simulink model "sampleModel7126_pp_1_1"  (R2018a)
settings: Solver=VariableStepAuto  StartTime=0.0  StopTime=10.0  RelTol=1e-3
undefined symbols (not defined in the file): DiscIntNeverNeededParam
libraries: simulink x367
(part 7 of 12)

== system sampleModel7126_pp_1_1/cfblk249/cfblk10 ==
  emi_1784 : Inport
  emi_1785 : Inport  Port=2
  Action Port : ActionPort  ActionType=then
  cfblk10 : simulink/Continuous/PID Controller (2DOF)  Controller=PID  TimeDomain=Discrete-time  SampleTime=-1  IntegratorMethod=Forward Euler  FilterMethod=Forward Euler  Form=Parallel  UseFilter=on  ControllerParametersSource=internal  P=1  I=1  D=0  N=100  b=1  c=1  InitialConditionSource=internal  InitialConditionForIntegrator=0  InitialConditionForFilter=0  ExternalReset=none  LimitOutput=off  UpperSaturationLimit=inf  LowerSaturationLimit=-inf  LinearizeAsGain=off  AntiWindupMode=none  Kb=1  TrackingMode=off  Kt=1  PParamMin=[]  PParamMax=[]  IParamMin=[]  IParamMax=[]  DParamMin=[]  DParamMax=[]  NParamMin=[]  NParamMax=[]  bParamMin=[]  bParamMax=[]  cParamMin=[]  cParamMax=[]  KbParamMin=[]  KbParamMax=[]  KtParamMin=[]  KtParamMax=[]  POutMin=[]  POutMax=[]  IOutMin=[]  IOutMax=[]  DOutMin=[]  DOutMax=[]  NOutMin=[]  NOutMax=[]  bOutMin=[]  bOutMax=[]  cOutMin=[]  cOutMax=[]  KbOutMin=[]  KbOutMax=[]  KtOutMin=[]  KtOutMax=[]  IntegratorOutMin=[]  IntegratorOutMax=[]  FilterOutMin=[]  FilterOutMax=[]  SumOutMin=[]  SumOutMax=[]  Sum1OutMin=[]  Sum1OutMax=[]  Sum2OutMin=[]  Sum2OutMax=[]  Sum3OutMin=[]  Sum3OutMax=[]  SumI1OutMin=[]  SumI1OutMax=[]  SumI2OutMin=[]  SumI2OutMax=[]  SumI3OutMin=[]  SumI3OutMax=[]  SumDOutMin=[]  SumDOutMax=[]  SaturationOutMin=[]  SaturationOutMax=[]  IntegratorContinuousStateAttributes=''  IntegratorStateMustResolveToSignalObject=off  IntegratorRTWStateStorageClass=Auto  FilterContinuousStateAttributes=''  FilterStateMustResolveToSignalObject=off  FilterRTWStateStorageClass=Auto  DifferentiatorICPrevScaledInput=0  DifferentiatorOutMin=[]  DifferentiatorOutMax=[]  FilterDiffOutCoefMin=[]  FilterDiffOutCoefMax=[]  SumDenOutMin=[]  SumDenOutMax=[]  SumNumOutMin=[]  SumNumOutMax=[]  ReciprocalOutMin=[]  ReciprocalOutMax=[]  DivideOutMin=[]  DivideOutMax=[]  TunerSelectOption=Transfer Function Based (PID Tuner App)
  emi_1786 : Outport
  wires:
  emi_1784/1 -> cfblk10/1
  emi_1785/1 -> cfblk10/2
  cfblk10/1 -> emi_1786/1

== system sampleModel7126_pp_1_1/cfblk249/cfblk3 ==
  emi_2116 : Inport
  Action Port : ActionPort  ActionType=then
  cfblk3 : DiscreteZeroPole  Poles=[0 0.5]  Gain=1  SampleTime=-1
  emi_2117 : Outport
  wires:
  emi_2116/1 -> cfblk3/1
  cfblk3/1 -> emi_2117/1

== system sampleModel7126_pp_1_1/cfblk249/cfblk5 ==
  emi_542 : Inport
  Action Port : ActionPort  ActionType=then
  cfblk5 : UnitDelay  SampleTime=-1
  emi_543 : Outport
  wires:
  emi_542/1 -> cfblk5/1
  cfblk5/1 -> emi_543/1

== system sampleModel7126_pp_1_1/cfblk249/cfblk9 ==
  emi_577 : Inport
  Action Port : ActionPort  ActionType=then
  cfblk9 : DiscreteFir
  emi_578 : Outport
  wires:
  emi_577/1 -> cfblk9/1
  cfblk9/1 -> emi_578/1

== system sampleModel7126_pp_1_1/cfblk249/emi_1787 ==
  Action Port : ActionPort  ActionType=else
  emi_1788 : Assertion

== system sampleModel7126_pp_1_1/cfblk249/emi_2118 ==
  Action Port : ActionPort  ActionType=else
  emi_2119 : Assertion

== system sampleModel7126_pp_1_1/cfblk249/emi_544 ==
  Action Port : ActionPort  ActionType=else
  emi_545 : Assertion

== system sampleModel7126_pp_1_1/cfblk249/emi_579 ==
  Action Port : ActionPort  ActionType=else
  emi_580 : Assertion

== system sampleModel7126_pp_1_1/cfblk250/cfblk4 ==
  emi_1841 : Inport
  Action Port : ActionPort  ActionType=then
  cfblk4 : simulink/Discrete/Transfer Fcn Real Zero  ZeroZ=0.75  ICPrevInput=0.0  DoSatur=off
      settings: SourceProductName=Simulink  SourceProductBaseCode=SL
  emi_1842 : Outport
  wires:
  emi_1841/1 -> cfblk4/1
  cfblk4/1 -> emi_1842/1

== system sampleModel7126_pp_1_1/cfblk250/cfblk6 ==
  emi_1313 : Inport
  Action Port : ActionPort  ActionType=then
  cfblk6 : DiscreteFir
  emi_1314 : Outport
  wires:
  emi_1313/1 -> cfblk6/1
  cfblk6/1 -> emi_1314/1

== system sampleModel7126_pp_1_1/cfblk250/emi_1315 ==
  Action Port : ActionPort  ActionType=else
  emi_1316 : Assertion

== system sampleModel7126_pp_1_1/cfblk250/emi_1843 ==
  Action Port : ActionPort  ActionType=else
  emi_1844 : Assertion

== system sampleModel7126_pp_1_1/cfblk251/cfblk5 ==
  emi_1490 : Inport
  Action Port : ActionPort  ActionType=then
  cfblk5 : simulink/Discrete/Transfer Fcn Real Zero  ZeroZ=0.75  ICPrevInput=0.0  DoSatur=off
      settings: SourceProductName=Simulink  SourceProductBaseCode=SL
  emi_1491 : Outport
  wires:
  emi_1490/1 -> cfblk5/1
  cfblk5/1 -> emi_1491/1

== system sampleModel7126_pp_1_1/cfblk251/cfblk6 ==
  emi_1398 : Inport
  Action Port : ActionPort  ActionType=then
  cfblk6 : simulink/Discrete/Transfer Fcn Lead or Lag  PoleZ=0.95  ZeroZ=0.75  ICPrevOutput=0.0  ICPrevInput=0.0  DoSatur=off
      settings: SourceProductName=Simulink  SourceProductBaseCode=SL
  emi_1399 : Outport
  wires:
  emi_1398/1 -> cfblk6/1
  cfblk6/1 -> emi_1399/1

== system sampleModel7126_pp_1_1/cfblk251/emi_1400 ==
  Action Port : ActionPort  ActionType=else
  emi_1401 : Assertion

== system sampleModel7126_pp_1_1/cfblk251/emi_1492 ==
  Action Port : ActionPort  ActionType=else
  emi_1493 : Assertion

== system sampleModel7126_pp_1_1/cfblk252/cfblk10 ==
  emi_1059 : Inport
  Action Port : ActionPort  ActionType=then
  cfblk10 : simulink/Discrete/Tapped Delay  vinit=0.0  samptime=-1  NumDelays=1  DelayOrder=Oldest  includeCurrent=off
  emi_1060 : Outport
  wires:
  emi_1059/1 -> cfblk10/1
  cfblk10/1 -> emi_1060/1

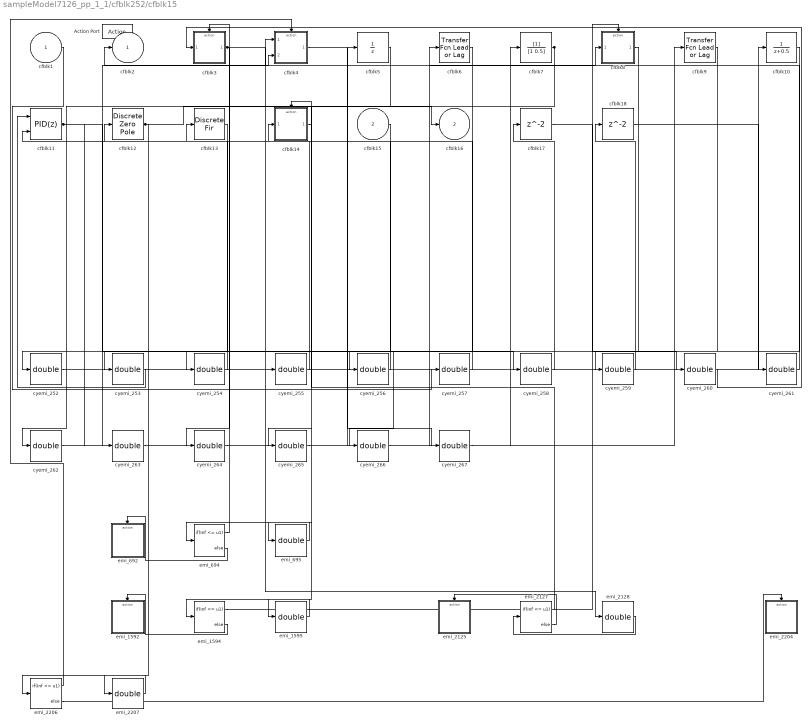
== system sampleModel7126_pp_1_1/cfblk252/cfblk15 ==
  cfblk1 : Inport
  cfblk15 : Inport  Port=2
  Action Port : ActionPort  ActionType=then
  cfblk10 : DiscreteTransferFcn
  cfblk11 : simulink/Continuous/PID Controller (2DOF)  Controller=PID  TimeDomain=Discrete-time  SampleTime=-1  IntegratorMethod=Forward Euler  FilterMethod=Forward Euler  Form=Parallel  UseFilter=on  ControllerParametersSource=internal  P=1  I=1  D=0  N=100  b=1  c=1  InitialConditionSource=internal  InitialConditionForIntegrator=0  InitialConditionForFilter=0  ExternalReset=none  LimitOutput=off  UpperSaturationLimit=inf  LowerSaturationLimit=-inf  LinearizeAsGain=off  AntiWindupMode=none  Kb=1  TrackingMode=off  Kt=1  PParamMin=[]  PParamMax=[]  IParamMin=[]  IParamMax=[]  DParamMin=[]  DParamMax=[]  NParamMin=[]  NParamMax=[]  bParamMin=[]  bParamMax=[]  cParamMin=[]  cParamMax=[]  KbParamMin=[]  KbParamMax=[]  KtParamMin=[]  KtParamMax=[]  POutMin=[]  POutMax=[]  IOutMin=[]  IOutMax=[]  DOutMin=[]  DOutMax=[]  NOutMin=[]  NOutMax=[]  bOutMin=[]  bOutMax=[]  cOutMin=[]  cOutMax=[]  KbOutMin=[]  KbOutMax=[]  KtOutMin=[]  KtOutMax=[]  IntegratorOutMin=[]  IntegratorOutMax=[]  FilterOutMin=[]  FilterOutMax=[]  SumOutMin=[]  SumOutMax=[]  Sum1OutMin=[]  Sum1OutMax=[]  Sum2OutMin=[]  Sum2OutMax=[]  Sum3OutMin=[]  Sum3OutMax=[]  SumI1OutMin=[]  SumI1OutMax=[]  SumI2OutMin=[]  SumI2OutMax=[]  SumI3OutMin=[]  SumI3OutMax=[]  SumDOutMin=[]  SumDOutMax=[]  SaturationOutMin=[]  SaturationOutMax=[]  IntegratorContinuousStateAttributes=''  IntegratorStateMustResolveToSignalObject=off  IntegratorRTWStateStorageClass=Auto  FilterContinuousStateAttributes=''  FilterStateMustResolveToSignalObject=off  FilterRTWStateStorageClass=Auto  DifferentiatorICPrevScaledInput=0  DifferentiatorOutMin=[]  DifferentiatorOutMax=[]  FilterDiffOutCoefMin=[]  FilterDiffOutCoefMax=[]  SumDenOutMin=[]  SumDenOutMax=[]  SumNumOutMin=[]  SumNumOutMax=[]  ReciprocalOutMin=[]  ReciprocalOutMax=[]  DivideOutMin=[]  DivideOutMax=[]  TunerSelectOption=Transfer Function Based (PID Tuner App)
  cfblk12 : DiscreteZeroPole  Poles=[0 0.5]  Gain=1  SampleTime=-1
  cfblk13 : DiscreteFir
  cfblk14 : Subsystem  TreatAsAtomicUnit=on
  cfblk17 : Delay
  cfblk18 : Delay
  cfblk3 : Subsystem  TreatAsAtomicUnit=on
  cfblk4 : Subsystem  TreatAsAtomicUnit=on
  cfblk5 : UnitDelay  SampleTime=-1
  cfblk6 : simulink/Discrete/Transfer Fcn Lead or Lag  PoleZ=0.95  ZeroZ=0.75  ICPrevOutput=0.0  ICPrevInput=0.0  DoSatur=off
      settings: SourceProductName=Simulink  SourceProductBaseCode=SL
  cfblk7 : DiscreteFilter
  cfblk8 : Subsystem  TreatAsAtomicUnit=on
  cfblk9 : simulink/Discrete/Transfer Fcn Lead or Lag  PoleZ=0.95  ZeroZ=0.75  ICPrevOutput=0.0  ICPrevInput=0.0  DoSatur=off
      settings: SourceProductName=Simulink  SourceProductBaseCode=SL
  cyemi_{252..267} (16 alike) : DataTypeConversion  OutDataTypeStr=double
  emi_1592 : Subsystem  TreatAsAtomicUnit=on
  emi_{694,1594,2127,2206} (4 alike) : If  IfExpression=Inf <= u1  SampleTime=[1 0]
  emi_{695,1595,2128,2207} (4 alike) : DataTypeConversion  OutDataTypeStr=double
  emi_2125 : Subsystem  TreatAsAtomicUnit=on
  emi_2204 : Subsystem  TreatAsAtomicUnit=on
  emi_692 : Subsystem  TreatAsAtomicUnit=on
  cfblk2 : Outport
  cfblk16 : Outport  Port=2
  wires:
  cfblk11/1 -> cyemi_258/1, cyemi_263/1
  cfblk12/1 -> cfblk16/1, emi_2207/1
  cfblk7/1 -> cfblk2/1, emi_695/1, emi_1595/1
  cyemi_252/1 -> cfblk10/1
  cfblk9/1 -> cyemi_252/1
  cyemi_253/1 -> cfblk11/1
  cfblk13/1 -> cyemi_253/1
  cyemi_254/1 -> cfblk11/2
  cyemi_255/1 -> cfblk12/1
  cyemi_256/1 -> cfblk13/1
  cfblk6/1 -> cyemi_256/1
  cfblk1/1 -> cyemi_257/1
  cyemi_258/1 -> cfblk17/1
  cyemi_259/1 -> cfblk18/1
  cfblk17/1 -> cyemi_260/1
  cfblk18/1 -> cyemi_261/1
  cfblk5/1 -> cyemi_262/1
  cyemi_263/1 -> cfblk5/1
  cyemi_264/1 -> cfblk6/1
  cfblk15/1 -> cyemi_264/1
  cyemi_265/1 -> cfblk7/1
  cfblk10/1 -> cyemi_266/1
  cyemi_267/1 -> cfblk9/1
  cyemi_260/1 -> cfblk3/1(emi_690)
  cfblk3/1(emi_691) -> cyemi_255/1, cyemi_254/1, emi_2128/1
  emi_694/1 -> cfblk3/Action
  emi_694/2 -> emi_692/Action
  emi_695/1 -> emi_694/1
  cyemi_266/1 -> cfblk8/1(emi_1590)
  cfblk8/1(emi_1591) -> cyemi_259/1
  emi_1594/1 -> cfblk8/Action
  emi_1594/2 -> emi_1592/Action
  emi_1595/1 -> emi_1594/1
  cyemi_257/1 -> cfblk14/1(emi_2123)
  cfblk14/1(emi_2124) -> cyemi_265/1
  emi_2127/1 -> cfblk14/Action
  emi_2127/2 -> emi_2125/Action
  emi_2128/1 -> emi_2127/1
  cyemi_261/1 -> cfblk4/1(emi_2201)
  cyemi_262/1 -> cfblk4/2(emi_2202)
  cfblk4/1(emi_2203) -> cyemi_267/1
  emi_2206/1 -> cfblk4/Action
  emi_2206/2 -> emi_2204/Action
  emi_2207/1 -> emi_2206/1

== system sampleModel7126_pp_1_1/cfblk252/cfblk16 ==
  cfblk1 : Inport
  cfblk16 : Inport  Port=2
  Action Port : ActionPort  ActionType=else
  cfblk10 : simulink/Discrete/Difference  ICPrevInput=0.0  OutMin=[]  OutMax=[]  OutDataTypeStr=double  OutputDataTypeScalingMode=double  OutDataType=fixdt(1, 16)  OutScaling=2^-10  DoSatur=off
  cfblk11 : DiscreteIntegrator  SampleTime=-1  OutDataTypeStr=double  ICPrevOutput=DiscIntNeverNeededParam  ICPrevScaledInput=DiscIntNeverNeededParam
  cfblk12 : simulink/Discrete/Transfer Fcn Real Zero  ZeroZ=0.75  ICPrevInput=0.0  DoSatur=off
      settings: SourceProductName=Simulink  SourceProductBaseCode=SL
  cfblk13 : Subsystem  TreatAsAtomicUnit=on
  cfblk14 : Delay  DelayLengthSource=Input port
      settings: InputPortMap=u0,p1
  cfblk15 : DiscreteFilter
  cfblk3 : Subsystem  TreatAsAtomicUnit=on
  cfblk4 : simulink/Discrete/Tapped Delay  vinit=0.0  samptime=-1  NumDelays=1  DelayOrder=Oldest  includeCurrent=off
  cfblk5 : simulink/Discrete/Transfer Fcn Lead or Lag  PoleZ=0.95  ZeroZ=0.75  ICPrevOutput=0.0  ICPrevInput=0.0  DoSatur=off
      settings: SourceProductName=Simulink  SourceProductBaseCode=SL
  cfblk6 : Delay  ShowEnablePort=on
      settings: InputPortMap=u0,e6
  cfblk7 : Subsystem  TreatAsAtomicUnit=on
  cfblk8 : simulink/Discrete/Transfer Fcn Lead or Lag  PoleZ=0.95  ZeroZ=0.75  ICPrevOutput=0.0  ICPrevInput=0.0  DoSatur=off
      settings: SourceProductName=Simulink  SourceProductBaseCode=SL
  cfblk9 : UnitDelay  SampleTime=-1
  cyemi_{270..285} (16 alike) : DataTypeConversion  OutDataTypeStr=double
  emi_1097 : Subsystem  TreatAsAtomicUnit=on
  emi_1099 : If  IfExpression=0 <= u1  SampleTime=[1 0]
  emi_1100 : DataTypeConversion  OutDataTypeStr=double
  emi_112 : Subsystem  TreatAsAtomicUnit=on
  emi_114 : If  IfExpression=0 <= u1  SampleTime=[1 0]
  emi_115 : DataTypeConversion  OutDataTypeStr=double
  emi_261 : Subsystem  TreatAsAtomicUnit=on
  emi_263 : If  IfExpression=0 <= u1  SampleTime=[1 0]
  emi_264 : DataTypeConversion  OutDataTypeStr=double
  cfblk2 : Outport
  cfblk17 : Outport  Port=2
  wires:
  cfblk8/1 -> cyemi_270/1, cyemi_281/1
  cfblk9/1 -> cfblk2/1
  cyemi_270/1 -> cfblk10/1
  cyemi_271/1 -> cfblk11/1
  cfblk4/1 -> cyemi_271/1, emi_115/1
  cyemi_272/1 -> cfblk12/1
  cfblk10/1 -> cyemi_273/1
  cyemi_274/1 -> cfblk14/1
  cfblk15/1 -> cyemi_274/1, cyemi_275/1
  cyemi_275/1 -> cfblk14/2
  cyemi_276/1 -> cfblk15/1
  cfblk5/1 -> cyemi_276/1
  cfblk14/1 -> cyemi_277/1
  cfblk16/1 -> cyemi_278/1
  cyemi_279/1 -> cfblk4/1
  cyemi_280/1 -> cfblk5/1
  cyemi_281/1 -> cfblk6/1
  cyemi_282/1 -> cfblk6/2
  cfblk12/1 -> cyemi_282/1
  cfblk1/1 -> cyemi_283/1
  cyemi_284/1 -> cfblk8/1
  cfblk11/1 -> cyemi_284/1
  cyemi_285/1 -> cfblk9/1
  cfblk6/1 -> cyemi_285/1
  cyemi_277/1 -> cfblk3/1(emi_109)
  cyemi_278/1 -> cfblk3/2(emi_110)
  cfblk3/1(emi_111) -> cyemi_279/1, emi_264/1, emi_1100/1
  emi_114/1 -> cfblk3/Action
  emi_114/2 -> emi_112/Action
  emi_115/1 -> emi_114/1
  cyemi_273/1 -> cfblk13/1(emi_259)
  cfblk13/1(emi_260) -> cyemi_272/1, cfblk17/1
  emi_263/1 -> cfblk13/Action
  emi_263/2 -> emi_261/Action
  emi_264/1 -> emi_263/1
  cyemi_283/1 -> cfblk7/1(emi_1095)
  cfblk7/1(emi_1096) -> cyemi_280/1
  emi_1099/1 -> cfblk7/Action
  emi_1099/2 -> emi_1097/Action
  emi_1100/1 -> emi_1099/1

== system sampleModel7126_pp_1_1/cfblk252/cfblk7 ==
  emi_166 : Inport
  Action Port : ActionPort  ActionType=then
  cfblk7 : UnitDelay  SampleTime=-1
  emi_167 : Outport
  wires:
  emi_166/1 -> cfblk7/1
  cfblk7/1 -> emi_167/1

== system sampleModel7126_pp_1_1/cfblk252/cfblk8 ==
  emi_2080 : Inport
  Action Port : ActionPort  ActionType=then
  cfblk8 : simulink/Discrete/Difference  ICPrevInput=0.0  OutMin=[]  OutMax=[]  OutDataTypeStr=double  OutputDataTypeScalingMode=double  OutDataType=fixdt(1, 16)  OutScaling=2^-10  DoSatur=off
  emi_2081 : Outport
  wires:
  emi_2080/1 -> cfblk8/1
  cfblk8/1 -> emi_2081/1

== system sampleModel7126_pp_1_1/cfblk252/emi_1061 ==
  Action Port : ActionPort  ActionType=else
  emi_1062 : Assertion

== system sampleModel7126_pp_1_1/cfblk252/emi_168 ==
  Action Port : ActionPort  ActionType=else
  emi_169 : Assertion

== system sampleModel7126_pp_1_1/cfblk252/emi_2082 ==
  Action Port : ActionPort  ActionType=else
  emi_2083 : Assertion

== system sampleModel7126_pp_1_1/cfblk253/cfblk10 ==
  cfblk1 : Inport
  cfblk12 : Inport  Port=2
  cfblk13 : Inport  Port=3
  cfblk14 : Inport  Port=4
  Action Port : ActionPort  ActionType=else
  cfblk10 : DiscreteFilter
  cfblk11 : Subsystem  TreatAsAtomicUnit=on
  cfblk3 : simulink/Discrete/Transfer Fcn First Order  PoleZ=0.95  ICPrevOutput=0.0  DoSatur=off
      settings: SourceProductName=Simulink
  cfblk4 : simulink/Discrete/Difference  ICPrevInput=0.0  OutMin=[]  OutMax=[]  OutDataTypeStr=double  OutputDataTypeScalingMode=double  OutDataType=fixdt(1, 16)  OutScaling=2^-10  DoSatur=off
  cfblk5 : DiscreteStateSpace  SampleTime=-1
  cfblk6 : Delay
  cfblk7 : DiscreteZeroPole  Poles=[0 0.5]  Gain=1  SampleTime=-1
  cfblk8 : Delay
  cfblk9 : UnitDelay  SampleTime=-1
  cyemi_{303..311} (9 alike) : DataTypeConversion  OutDataTypeStr=double
  emi_2111 : Subsystem  TreatAsAtomicUnit=on
  emi_2113 : If  IfExpression=0 <= u1  SampleTime=[1 0]
  emi_2114 : DataTypeConversion  OutDataTypeStr=double
  cfblk2 : Outport
  cfblk15 : Outport  Port=2
  wires:
  cfblk3/1 -> cfblk2/1
  cfblk12/1 -> cfblk15/1
  cyemi_303/1 -> cfblk10/1
  cfblk8/1 -> cyemi_303/1
  cfblk10/1 -> cyemi_304/1
  cyemi_305/1 -> cfblk3/1
  cfblk7/1 -> cyemi_305/1
  cyemi_306/1 -> cfblk4/1
  cfblk5/1 -> cyemi_306/1, emi_2114/1
  cyemi_307/1 -> cfblk5/1
  cfblk14/1 -> cyemi_307/1
  cyemi_308/1 -> cfblk6/1
  cfblk1/1 -> cyemi_308/1
  cyemi_309/1 -> cfblk7/1
  cyemi_310/1 -> cfblk8/1
  cfblk13/1 -> cyemi_310/1
  cyemi_311/1 -> cfblk9/1
  cfblk4/1 -> cyemi_311/1
  cyemi_304/1 -> cfblk11/1(emi_2109)
  cfblk11/1(emi_2110) -> cyemi_309/1
  emi_2113/1 -> cfblk11/Action
  emi_2113/2 -> emi_2111/Action
  emi_2114/1 -> emi_2113/1

== system sampleModel7126_pp_1_1/cfblk253/cfblk15 ==
  emi_711 : Inport
  Action Port : ActionPort  ActionType=then
  cfblk15 : Delay
  emi_712 : Outport
  wires:
  emi_711/1 -> cfblk15/1
  cfblk15/1 -> emi_712/1

== system sampleModel7126_pp_1_1/cfblk253/cfblk4 ==
  emi_1497 : Inport
  Action Port : ActionPort  ActionType=then
  cfblk4 : simulink/Discrete/Transfer Fcn Real Zero  ZeroZ=0.75  ICPrevInput=0.0  DoSatur=off
      settings: SourceProductName=Simulink  SourceProductBaseCode=SL
  emi_1498 : Outport
  wires:
  emi_1497/1 -> cfblk4/1
  cfblk4/1 -> emi_1498/1

== system sampleModel7126_pp_1_1/cfblk253/cfblk9 ==
  cfblk1 : Inport
  cfblk4 : Inport  Port=2
  cfblk5 : Inport  Port=3
  cfblk6 : Inport  Port=4
  Action Port : ActionPort  ActionType=then
  cfblk3 : DiscreteZeroPole  Poles=[0 0.5]  Gain=1  SampleTime=-1
  cyemi_327 : DataTypeConversion  OutDataTypeStr=double
  cfblk2 : Outport
  cfblk7 : Outport  Port=2
  cfblk8 : Outport  Port=3
  cfblk9 : Outport  Port=4
  wires:
  cfblk1/1 -> cfblk2/1
  cfblk6/1 -> cfblk8/1
  cfblk5/1 -> cfblk7/1
  cfblk3/1 -> cfblk9/1
  cyemi_327/1 -> cfblk3/1
  cfblk4/1 -> cyemi_327/1

== system sampleModel7126_pp_1_1/cfblk253/emi_1499 ==
  Action Port : ActionPort  ActionType=else
  emi_1500 : Assertion

== system sampleModel7126_pp_1_1/cfblk253/emi_713 ==
  Action Port : ActionPort  ActionType=else
  emi_714 : Assertion

== system sampleModel7126_pp_1_1/cfblk255/cfblk3 ==
  emi_774 : Inport
  Action Port : ActionPort  ActionType=then
  cfblk3 : simulink/Discrete/Transfer Fcn Lead or Lag  PoleZ=0.95  ZeroZ=0.75  ICPrevOutput=0.0  ICPrevInput=0.0  DoSatur=off
      settings: SourceProductName=Simulink  SourceProductBaseCode=SL
  emi_775 : Outport
  wires:
  emi_774/1 -> cfblk3/1
  cfblk3/1 -> emi_775/1

== system sampleModel7126_pp_1_1/cfblk255/cfblk5 ==
  emi_1792 : Inport
  Action Port : ActionPort  ActionType=then
  cfblk5 : Delay
  emi_1793 : Outport
  wires:
  emi_1792/1 -> cfblk5/1
  cfblk5/1 -> emi_1793/1

== system sampleModel7126_pp_1_1/cfblk255/cfblk6 ==
  emi_945 : Inport
  emi_946 : Inport  Port=2
  Action Port : ActionPort  ActionType=then
  cfblk6 : Delay  ShowEnablePort=on
      settings: InputPortMap=u0,e6
  emi_947 : Outport
  wires:
  emi_945/1 -> cfblk6/1
  emi_946/1 -> cfblk6/2
  cfblk6/1 -> emi_947/1

== system sampleModel7126_pp_1_1/cfblk255/emi_1794 ==
  Action Port : ActionPort  ActionType=else
  emi_1795 : Assertion

== system sampleModel7126_pp_1_1/cfblk255/emi_776 ==
  Action Port : ActionPort  ActionType=else
  emi_777 : Assertion

== system sampleModel7126_pp_1_1/cfblk255/emi_948 ==
  Action Port : ActionPort  ActionType=else
  emi_949 : Assertion

== system sampleModel7126_pp_1_1/cfblk256/cfblk11 ==
  cfblk1 : Inport
  cfblk9 : Inport  Port=2
  cfblk10 : Inport  Port=3
  Action Port : ActionPort  ActionType=then
  cfblk3 : Subsystem  TreatAsAtomicUnit=on
  cfblk4 : simulink/Discrete/Transfer Fcn Real Zero  ZeroZ=0.75  ICPrevInput=0.0  DoSatur=off
      settings: SourceProductName=Simulink  SourceProductBaseCode=SL
  cfblk5 : DiscreteStateSpace  SampleTime=-1
  cfblk6 : DiscreteTransferFcn
  cfblk7 : Subsystem  TreatAsAtomicUnit=on
  cfblk8 : DiscreteFir
  cyemi_{362..367} (6 alike) : DataTypeConversion  OutDataTypeStr=double
  emi_1133 : Subsystem  TreatAsAtomicUnit=on
  emi_1135 : If  IfExpression=Inf <= u1
  emi_1136 : DataTypeConversion  OutDataTypeStr=double
  emi_572 : Subsystem  TreatAsAtomicUnit=on
  emi_574 : If  IfExpression=Inf <= u1  SampleTime=[1 0]
  emi_575 : DataTypeConversion  OutDataTypeStr=double
  cfblk2 : Outport
  cfblk11 : Outport  Port=2
  wires:
  cfblk6/1 -> cfblk11/1, emi_1136/1
  cfblk9/1 -> cyemi_362/1
  cyemi_363/1 -> cfblk4/1
  cfblk1/1 -> cyemi_363/1
  cyemi_364/1 -> cfblk5/1
  cfblk8/1 -> cyemi_364/1
  cyemi_365/1 -> cfblk6/1
  cfblk4/1 -> cyemi_365/1
  cfblk5/1 -> cyemi_366/1, emi_575/1
  cyemi_367/1 -> cfblk8/1
  cyemi_366/1 -> cfblk7/1(emi_570)
  cfblk7/1(emi_571) -> cfblk2/1
  emi_574/1 -> cfblk7/Action
  emi_574/2 -> emi_572/Action
  emi_575/1 -> emi_574/1
  cyemi_362/1 -> cfblk3/1(emi_1131)
  cfblk3/1(emi_1132) -> cyemi_367/1
  emi_1135/1 -> cfblk3/Action
  emi_1135/2 -> emi_1133/Action
  emi_1136/1 -> emi_1135/1

== system sampleModel7126_pp_1_1/cfblk256/cfblk12 ==
  cfblk1 : Inport
  Action Port : ActionPort  ActionType=else
  cfblk3 : DiscreteTransferFcn
  cfblk4 : simulink/Discrete/Difference  ICPrevInput=0.0  OutMin=[]  OutMax=[]  OutDataTypeStr=double  OutputDataTypeScalingMode=double  OutDataType=fixdt(1, 16)  OutScaling=2^-10  DoSatur=off
  cfblk5 : DiscreteIntegrator  SampleTime=-1  OutDataTypeStr=double  ICPrevOutput=DiscIntNeverNeededParam  ICPrevScaledInput=DiscIntNeverNeededParam
  cfblk6 : Delay
  cyemi_{369..372} (4 alike) : DataTypeConversion  OutDataTypeStr=double
  cfblk2 : Outport
  cfblk7 : Outport  Port=2
  cfblk8 : Outport  Port=3
  wires:
  cfblk4/1 -> cfblk7/1, cfblk2/1
  cfblk3/1 -> cfblk8/1, cyemi_371/1
  cyemi_369/1 -> cfblk3/1
  cfblk1/1 -> cyemi_369/1
  cyemi_370/1 -> cfblk4/1
  cfblk6/1 -> cyemi_370/1
  cyemi_371/1 -> cfblk5/1
  cyemi_372/1 -> cfblk6/1
  cfblk5/1 -> cyemi_372/1

== system sampleModel7126_pp_1_1/cfblk256/cfblk14 ==
  emi_2144 : Inport
  Action Port : ActionPort  ActionType=then
  cfblk14 : Delay
  emi_2145 : Outport
  wires:
  emi_2144/1 -> cfblk14/1
  cfblk14/1 -> emi_2145/1

== system sampleModel7126_pp_1_1/cfblk256/cfblk3 ==
  emi_1038 : Inport
  Action Port : ActionPort  ActionType=then
  cfblk3 : DiscreteTransferFcn
  emi_1039 : Outport
  wires:
  emi_1038/1 -> cfblk3/1
  cfblk3/1 -> emi_1039/1

== system sampleModel7126_pp_1_1/cfblk256/emi_1040 ==
  Action Port : ActionPort  ActionType=else
  emi_1041 : Assertion

== system sampleModel7126_pp_1_1/cfblk256/emi_2146 ==
  Action Port : ActionPort  ActionType=else
  emi_2147 : Assertion

== system sampleModel7126_pp_1_1/cfblk257/cfblk7 ==
  emi_1632 : Inport
  Action Port : ActionPort  ActionType=then
  cfblk7 : simulink/Continuous/PID Controller  Controller=PID  TimeDomain=Discrete-time  SampleTime=-1  IntegratorMethod=Forward Euler  FilterMethod=Forward Euler  Form=Parallel  UseFilter=on  ControllerParametersSource=internal  P=1  I=1  D=0  N=100  InitialConditionSource=internal  InitialConditionForIntegrator=0  InitialConditionForFilter=0  ExternalReset=none  LimitOutput=off  UpperSaturationLimit=inf  LowerSaturationLimit=-inf  LinearizeAsGain=off  AntiWindupMode=none  Kb=1  TrackingMode=off  Kt=1  PParamMin=[]  PParamMax=[]  IParamMin=[]  IParamMax=[]  DParamMin=[]  DParamMax=[]  NParamMin=[]  NParamMax=[]  KbParamMin=[]  KbParamMax=[]  KtParamMin=[]  KtParamMax=[]  POutMin=[]  POutMax=[]  IOutMin=[]  IOutMax=[]  DOutMin=[]  DOutMax=[]  NOutMin=[]  NOutMax=[]  KbOutMin=[]  KbOutMax=[]  KtOutMin=[]  KtOutMax=[]  IntegratorOutMin=[]  IntegratorOutMax=[]  FilterOutMin=[]  FilterOutMax=[]  SumOutMin=[]  SumOutMax=[]  SumI1OutMin=[]  SumI1OutMax=[]  SumI2OutMin=[]  SumI2OutMax=[]  SumI3OutMin=[]  SumI3OutMax=[]  SumDOutMin=[]  SumDOutMax=[]  SaturationOutMin=[]  SaturationOutMax=[]  IntegratorContinuousStateAttributes=''  IntegratorStateMustResolveToSignalObject=off  IntegratorRTWStateStorageClass=Auto  FilterContinuousStateAttributes=''  FilterStateMustResolveToSignalObject=off  FilterRTWStateStorageClass=Auto  DifferentiatorICPrevScaledInput=0  DifferentiatorOutMin=[]  DifferentiatorOutMax=[]  FilterDiffOutCoefMin=[]  FilterDiffOutCoefMax=[]  SumDenOutMin=[]  SumDenOutMax=[]  SumNumOutMin=[]  SumNumOutMax=[]  ReciprocalOutMin=[]  ReciprocalOutMax=[]  DivideOutMin=[]  DivideOutMax=[]  TunerSelectOption=Transfer Function Based (PID Tuner App)
  emi_1633 : Outport
  wires:
  emi_1632/1 -> cfblk7/1
  cfblk7/1 -> emi_1633/1

== system sampleModel7126_pp_1_1/cfblk257/cfblk9 ==
  emi_725 : Inport
  Action Port : ActionPort  ActionType=then
  cfblk9 : DiscreteStateSpace  SampleTime=-1
  emi_726 : Outport
  wires:
  emi_725/1 -> cfblk9/1
  cfblk9/1 -> emi_726/1

== system sampleModel7126_pp_1_1/cfblk257/emi_1634 ==
  Action Port : ActionPort  ActionType=else
  emi_1635 : Assertion

== system sampleModel7126_pp_1_1/cfblk257/emi_727 ==
  Action Port : ActionPort  ActionType=else
  emi_728 : Assertion

== system sampleModel7126_pp_1_1/cfblk258/cfblk5 ==
  emi_1341 : Inport
  Action Port : ActionPort  ActionType=then
  cfblk5 : UnitDelay  SampleTime=-1
  emi_1342 : Outport
  wires:
  emi_1341/1 -> cfblk5/1
  cfblk5/1 -> emi_1342/1

== system sampleModel7126_pp_1_1/cfblk258/emi_1343 ==
  Action Port : ActionPort  ActionType=else
  emi_1344 : Assertion

== system sampleModel7126_pp_1_1/cfblk259/cfblk10 ==
  cfblk1 : Inport
  cfblk10 : Inport  Port=2
  cfblk11 : Inport  Port=3
  cfblk12 : Inport  Port=4
  Action Port : ActionPort  ActionType=else
  cfblk13 : Subsystem  TreatAsAtomicUnit=on
  cfblk3 : DiscreteZeroPole  Poles=[0 0.5]  Gain=1  SampleTime=-1
  cfblk4 : Subsystem  TreatAsAtomicUnit=on
  cfblk5 : DiscreteStateSpace  SampleTime=-1
  cfblk6 : Subsystem  TreatAsAtomicUnit=on
  cfblk7 : DiscreteStateSpace  SampleTime=-1
  cfblk8 : simulink/Discrete/Transfer Fcn First Order  PoleZ=0.95  ICPrevOutput=0.0  DoSatur=off
      settings: SourceProductName=Simulink
  cfblk9 : Subsystem  TreatAsAtomicUnit=on
  cyemi_{412..420} (9 alike) : DataTypeConversion  OutDataTypeStr=double
  emi_1550 : Subsystem  TreatAsAtomicUnit=on
  emi_1552 : If  IfExpression=Inf <= u1  SampleTime=[1 0]
  emi_{377,816,865,1553} (4 alike) : DataTypeConversion  OutDataTypeStr=double
  emi_374 : Subsystem  TreatAsAtomicUnit=on
  emi_376 : If  IfExpression=Inf <= u1
  emi_813 : Subsystem  TreatAsAtomicUnit=on
  emi_815 : If  IfExpression=Inf <= u1  SampleTime=[1 0]
  emi_862 : Subsystem  TreatAsAtomicUnit=on
  emi_864 : If  IfExpression=Inf <= u1  SampleTime=[1 0]
  cfblk2 : Outport
  wires:
  cfblk10/1 -> cfblk2/1
  cyemi_413/1 -> cfblk3/1
  cfblk5/1 -> cyemi_413/1, emi_377/1
  cfblk12/1 -> cyemi_414/1
  cyemi_416/1 -> cfblk5/1
  cfblk11/1 -> cyemi_416/1
  cyemi_418/1 -> cfblk7/1
  cyemi_419/1 -> cfblk8/1
  cfblk3/1 -> cyemi_419/1
  cfblk1/1 -> cyemi_420/1
  cyemi_412/1 -> cfblk13/1(emi_372)
  cfblk13/1(emi_373) -> cyemi_415/1, emi_816/1, emi_865/1
  emi_376/1 -> cfblk13/Action
  emi_376/2 -> emi_374/Action
  emi_377/1 -> emi_376/1
  cyemi_417/1 -> cfblk6/1(emi_811)
  cfblk6/1(emi_812) -> cyemi_412/1, emi_1553/1
  emi_815/1 -> cfblk6/Action
  emi_815/2 -> emi_813/Action
  emi_816/1 -> emi_815/1
  cyemi_420/1 -> cfblk9/1(emi_860)
  cfblk9/1(emi_861) -> cyemi_418/1
  emi_864/1 -> cfblk9/Action
  emi_864/2 -> emi_862/Action
  emi_865/1 -> emi_864/1
  cyemi_414/1 -> cfblk4/1(emi_1547)
  cyemi_415/1 -> cfblk4/2(emi_1548)
  cfblk4/1(emi_1549) -> cyemi_417/1
  emi_1552/1 -> cfblk4/Action
  emi_1552/2 -> emi_1550/Action
  emi_1553/1 -> emi_1552/1

== system sampleModel7126_pp_1_1/cfblk259/cfblk11 ==
  emi_43 : Inport
  Action Port : ActionPort  ActionType=then
  cfblk11 : Delay
  emi_44 : Outport
  wires:
  emi_43/1 -> cfblk11/1
  cfblk11/1 -> emi_44/1

== system sampleModel7126_pp_1_1/cfblk259/cfblk13 ==
  emi_58 : Inport
  Action Port : ActionPort  ActionType=then
  cfblk13 : Delay
  emi_59 : Outport
  wires:
  emi_58/1 -> cfblk13/1
  cfblk13/1 -> emi_59/1

== system sampleModel7126_pp_1_1/cfblk259/cfblk3 ==
  emi_1769 : Inport
  emi_1770 : Inport  Port=2
  Action Port : ActionPort  ActionType=then
  cfblk3 : Delay  DelayLengthSource=Input port
      settings: InputPortMap=u0,p1
  emi_1771 : Outport
  wires:
  emi_1769/1 -> cfblk3/1
  emi_1770/1 -> cfblk3/2
  cfblk3/1 -> emi_1771/1

== system sampleModel7126_pp_1_1/cfblk259/cfblk4 ==
  emi_1159 : Inport
  Action Port : ActionPort  ActionType=then
  cfblk4 : DiscreteFir
  emi_1160 : Outport
  wires:
  emi_1159/1 -> cfblk4/1
  cfblk4/1 -> emi_1160/1

== system sampleModel7126_pp_1_1/cfblk259/cfblk6 ==
  emi_556 : Inport
  Action Port : ActionPort  ActionType=then
  cfblk6 : simulink/Continuous/PID Controller  Controller=PID  TimeDomain=Discrete-time  SampleTime=-1  IntegratorMethod=Forward Euler  FilterMethod=Forward Euler  Form=Parallel  UseFilter=on  ControllerParametersSource=internal  P=1  I=1  D=0  N=100  InitialConditionSource=internal  InitialConditionForIntegrator=0  InitialConditionForFilter=0  ExternalReset=none  LimitOutput=off  UpperSaturationLimit=inf  LowerSaturationLimit=-inf  LinearizeAsGain=off  AntiWindupMode=none  Kb=1  TrackingMode=off  Kt=1  PParamMin=[]  PParamMax=[]  IParamMin=[]  IParamMax=[]  DParamMin=[]  DParamMax=[]  NParamMin=[]  NParamMax=[]  KbParamMin=[]  KbParamMax=[]  KtParamMin=[]  KtParamMax=[]  POutMin=[]  POutMax=[]  IOutMin=[]  IOutMax=[]  DOutMin=[]  DOutMax=[]  NOutMin=[]  NOutMax=[]  KbOutMin=[]  KbOutMax=[]  KtOutMin=[]  KtOutMax=[]  IntegratorOutMin=[]  IntegratorOutMax=[]  FilterOutMin=[]  FilterOutMax=[]  SumOutMin=[]  SumOutMax=[]  SumI1OutMin=[]  SumI1OutMax=[]  SumI2OutMin=[]  SumI2OutMax=[]  SumI3OutMin=[]  SumI3OutMax=[]  SumDOutMin=[]  SumDOutMax=[]  SaturationOutMin=[]  SaturationOutMax=[]  IntegratorContinuousStateAttributes=''  IntegratorStateMustResolveToSignalObject=off  IntegratorRTWStateStorageClass=Auto  FilterContinuousStateAttributes=''  FilterStateMustResolveToSignalObject=off  FilterRTWStateStorageClass=Auto  DifferentiatorICPrevScaledInput=0  DifferentiatorOutMin=[]  DifferentiatorOutMax=[]  FilterDiffOutCoefMin=[]  FilterDiffOutCoefMax=[]  SumDenOutMin=[]  SumDenOutMax=[]  SumNumOutMin=[]  SumNumOutMax=[]  ReciprocalOutMin=[]  ReciprocalOutMax=[]  DivideOutMin=[]  DivideOutMax=[]  TunerSelectOption=Transfer Function Based (PID Tuner App)
  emi_557 : Outport
  wires:
  emi_556/1 -> cfblk6/1
  cfblk6/1 -> emi_557/1

== system sampleModel7126_pp_1_1/cfblk259/cfblk9 ==
  cfblk1 : Inport
  cfblk11 : Inport  Port=2
  Action Port : ActionPort  ActionType=then
  cfblk10 : Subsystem  TreatAsAtomicUnit=on
  cfblk14 : Subsystem  TreatAsAtomicUnit=on
  cfblk15 : Delay
  cfblk3 : simulink/Discrete/Tapped Delay  vinit=0.0  samptime=-1  NumDelays=1  DelayOrder=Oldest  includeCurrent=off
  cfblk4 : Delay  ShowEnablePort=on
      settings: InputPortMap=u0,e6
  cfblk5 : simulink/Discrete/Transfer Fcn First Order  PoleZ=0.95  ICPrevOutput=0.0  DoSatur=off
      settings: SourceProductName=Simulink
  cfblk6 : DiscreteFilter
  cfblk7 : Delay  DelayLengthSource=Input port
      settings: InputPortMap=u0,p1
  cfblk8 : Subsystem  TreatAsAtomicUnit=on
  cfblk9 : Subsystem  TreatAsAtomicUnit=on
  cyemi_{432..445} (14 alike) : DataTypeConversion  OutDataTypeStr=double
  emi_1147 : Subsystem  TreatAsAtomicUnit=on
  emi_1149 : If  IfExpression=Inf <= u1
  emi_{406,1150,1289,1897} (4 alike) : DataTypeConversion  OutDataTypeStr=double
  emi_1286 : Subsystem  TreatAsAtomicUnit=on
  emi_1288 : If  IfExpression=Inf <= u1  SampleTime=[1 0]
  emi_1894 : Subsystem  TreatAsAtomicUnit=on
  emi_1896 : If  IfExpression=Inf <= u1  SampleTime=[1 0]
  emi_403 : Subsystem  TreatAsAtomicUnit=on
  emi_405 : If  IfExpression=Inf <= u1  SampleTime=[1 0]
  cfblk2 : Outport
  cfblk12 : Outport  Port=2
  cfblk13 : Outport  Port=3
  wires:
  cfblk6/1 -> cyemi_434/1, cyemi_438/1, emi_406/1
  cfblk3/1 -> cfblk2/1, cyemi_439/1
  cfblk7/1 -> cyemi_433/1
  cyemi_434/1 -> cfblk15/1
  cyemi_435/1 -> cfblk3/1
  cyemi_436/1 -> cfblk4/1
  cyemi_437/1 -> cfblk4/2
  cyemi_438/1 -> cfblk5/1
  cyemi_439/1 -> cfblk6/1
  cyemi_440/1 -> cfblk7/1
  cfblk5/1 -> cyemi_440/1
  cyemi_441/1 -> cfblk7/2
  cfblk4/1 -> cyemi_442/1
  cfblk15/1 -> cyemi_443/1
  cfblk11/1 -> cyemi_444/1
  cfblk1/1 -> cyemi_445/1
  cyemi_442/1 -> cfblk8/1(emi_400)
  cyemi_443/1 -> cfblk8/2(emi_401)
  cfblk8/1(emi_402) -> cyemi_432/1, cfblk13/1, cfblk12/1, emi_1897/1
  emi_405/1 -> cfblk8/Action
  emi_405/2 -> emi_403/Action
  emi_406/1 -> emi_405/1
  cyemi_432/1 -> cfblk10/1(emi_1145)
  cfblk10/1(emi_1146) -> cyemi_441/1, cyemi_435/1
  emi_1149/1 -> cfblk10/Action
  emi_1149/2 -> emi_1147/Action
  emi_1150/1 -> emi_1149/1
  cyemi_444/1 -> cfblk9/1(emi_1283)
  cyemi_445/1 -> cfblk9/2(emi_1284)
  cfblk9/1(emi_1285) -> cyemi_437/1
  emi_1288/1 -> cfblk9/Action
  emi_1288/2 -> emi_1286/Action
  emi_1289/1 -> emi_1288/1
  cyemi_433/1 -> cfblk14/1(emi_1892)
  cfblk14/1(emi_1893) -> emi_1289/1, emi_1150/1, cyemi_436/1
  emi_1896/1 -> cfblk14/Action
  emi_1896/2 -> emi_1894/Action
  emi_1897/1 -> emi_1896/1

== system sampleModel7126_pp_1_1/cfblk259/emi_1161 ==
  Action Port : ActionPort  ActionType=else
  emi_1162 : Assertion

== system sampleModel7126_pp_1_1/cfblk259/emi_1772 ==
  Action Port : ActionPort  ActionType=else
  emi_1773 : Assertion

== system sampleModel7126_pp_1_1/cfblk259/emi_45 ==
  Action Port : ActionPort  ActionType=else
  emi_46 : Assertion

== system sampleModel7126_pp_1_1/cfblk259/emi_558 ==
  Action Port : ActionPort  ActionType=else
  emi_559 : Assertion

== system sampleModel7126_pp_1_1/cfblk259/emi_60 ==
  Action Port : ActionPort  ActionType=else
  emi_61 : Assertion

== system sampleModel7126_pp_1_1/cfblk260/cfblk4 ==
  emi_252 : Inport
  Action Port : ActionPort  ActionType=then
  cfblk4 : simulink/Continuous/PID Controller  Controller=PID  TimeDomain=Discrete-time  SampleTime=-1  IntegratorMethod=Forward Euler  FilterMethod=Forward Euler  Form=Parallel  UseFilter=on  ControllerParametersSource=internal  P=1  I=1  D=0  N=100  InitialConditionSource=internal  InitialConditionForIntegrator=0  InitialConditionForFilter=0  ExternalReset=none  LimitOutput=off  UpperSaturationLimit=inf  LowerSaturationLimit=-inf  LinearizeAsGain=off  AntiWindupMode=none  Kb=1  TrackingMode=off  Kt=1  PParamMin=[]  PParamMax=[]  IParamMin=[]  IParamMax=[]  DParamMin=[]  DParamMax=[]  NParamMin=[]  NParamMax=[]  KbParamMin=[]  KbParamMax=[]  KtParamMin=[]  KtParamMax=[]  POutMin=[]  POutMax=[]  IOutMin=[]  IOutMax=[]  DOutMin=[]  DOutMax=[]  NOutMin=[]  NOutMax=[]  KbOutMin=[]  KbOutMax=[]  KtOutMin=[]  KtOutMax=[]  IntegratorOutMin=[]  IntegratorOutMax=[]  FilterOutMin=[]  FilterOutMax=[]  SumOutMin=[]  SumOutMax=[]  SumI1OutMin=[]  SumI1OutMax=[]  SumI2OutMin=[]  SumI2OutMax=[]  SumI3OutMin=[]  SumI3OutMax=[]  SumDOutMin=[]  SumDOutMax=[]  SaturationOutMin=[]  SaturationOutMax=[]  IntegratorContinuousStateAttributes=''  IntegratorStateMustResolveToSignalObject=off  IntegratorRTWStateStorageClass=Auto  FilterContinuousStateAttributes=''  FilterStateMustResolveToSignalObject=off  FilterRTWStateStorageClass=Auto  DifferentiatorICPrevScaledInput=0  DifferentiatorOutMin=[]  DifferentiatorOutMax=[]  FilterDiffOutCoefMin=[]  FilterDiffOutCoefMax=[]  SumDenOutMin=[]  SumDenOutMax=[]  SumNumOutMin=[]  SumNumOutMax=[]  ReciprocalOutMin=[]  ReciprocalOutMax=[]  DivideOutMin=[]  DivideOutMax=[]  TunerSelectOption=Transfer Function Based (PID Tuner App)
  emi_253 : Outport
  wires:
  emi_252/1 -> cfblk4/1
  cfblk4/1 -> emi_253/1

== system sampleModel7126_pp_1_1/cfblk260/cfblk5 ==
  emi_8 : Inport
  Action Port : ActionPort  ActionType=then
  cfblk5 : DiscreteIntegrator  SampleTime=-1  OutDataTypeStr=double  ICPrevOutput=DiscIntNeverNeededParam  ICPrevScaledInput=DiscIntNeverNeededParam
  emi_9 : Outport
  wires:
  emi_8/1 -> cfblk5/1
  cfblk5/1 -> emi_9/1

== system sampleModel7126_pp_1_1/cfblk260/cfblk6 ==
  emi_408 : Inport
  Action Port : ActionPort  ActionType=then
  cfblk6 : Delay
  emi_409 : Outport
  wires:
  emi_408/1 -> cfblk6/1
  cfblk6/1 -> emi_409/1

== system sampleModel7126_pp_1_1/cfblk260/emi_10 ==
  Action Port : ActionPort  ActionType=else
  emi_11 : Assertion

== system sampleModel7126_pp_1_1/cfblk260/emi_254 ==
  Action Port : ActionPort  ActionType=else
  emi_255 : Assertion

== system sampleModel7126_pp_1_1/cfblk260/emi_410 ==
  Action Port : ActionPort  ActionType=else
  emi_411 : Assertion

== system sampleModel7126_pp_1_1/cfblk261/cfblk13 ==
  cfblk1 : Inport
  Action Port : ActionPort  ActionType=then
  cfblk3 : simulink/Continuous/PID Controller (2DOF)  Controller=PID  TimeDomain=Discrete-time  SampleTime=-1  IntegratorMethod=Forward Euler  FilterMethod=Forward Euler  Form=Parallel  UseFilter=on  ControllerParametersSource=internal  P=1  I=1  D=0  N=100  b=1  c=1  InitialConditionSource=internal  InitialConditionForIntegrator=0  InitialConditionForFilter=0  ExternalReset=none  LimitOutput=off  UpperSaturationLimit=inf  LowerSaturationLimit=-inf  LinearizeAsGain=off  AntiWindupMode=none  Kb=1  TrackingMode=off  Kt=1  PParamMin=[]  PParamMax=[]  IParamMin=[]  IParamMax=[]  DParamMin=[]  DParamMax=[]  NParamMin=[]  NParamMax=[]  bParamMin=[]  bParamMax=[]  cParamMin=[]  cParamMax=[]  KbParamMin=[]  KbParamMax=[]  KtParamMin=[]  KtParamMax=[]  POutMin=[]  POutMax=[]  IOutMin=[]  IOutMax=[]  DOutMin=[]  DOutMax=[]  NOutMin=[]  NOutMax=[]  bOutMin=[]  bOutMax=[]  cOutMin=[]  cOutMax=[]  KbOutMin=[]  KbOutMax=[]  KtOutMin=[]  KtOutMax=[]  IntegratorOutMin=[]  IntegratorOutMax=[]  FilterOutMin=[]  FilterOutMax=[]  SumOutMin=[]  SumOutMax=[]  Sum1OutMin=[]  Sum1OutMax=[]  Sum2OutMin=[]  Sum2OutMax=[]  Sum3OutMin=[]  Sum3OutMax=[]  SumI1OutMin=[]  SumI1OutMax=[]  SumI2OutMin=[]  SumI2OutMax=[]  SumI3OutMin=[]  SumI3OutMax=[]  SumDOutMin=[]  SumDOutMax=[]  SaturationOutMin=[]  SaturationOutMax=[]  IntegratorContinuousStateAttributes=''  IntegratorStateMustResolveToSignalObject=off  IntegratorRTWStateStorageClass=Auto  FilterContinuousStateAttributes=''  FilterStateMustResolveToSignalObject=off  FilterRTWStateStorageClass=Auto  DifferentiatorICPrevScaledInput=0  DifferentiatorOutMin=[]  DifferentiatorOutMax=[]  FilterDiffOutCoefMin=[]  FilterDiffOutCoefMax=[]  SumDenOutMin=[]  SumDenOutMax=[]  SumNumOutMin=[]  SumNumOutMax=[]  ReciprocalOutMin=[]  ReciprocalOutMax=[]  DivideOutMin=[]  DivideOutMax=[]  TunerSelectOption=Transfer Function Based (PID Tuner App)
  cfblk4 : DiscreteFir
  cfblk5 : UnitDelay  SampleTime=-1
  cfblk6 : Delay  ShowEnablePort=on
      settings: InputPortMap=u0,e6
  cfblk7 : Subsystem  TreatAsAtomicUnit=on
  cfblk8 : Delay
  cyemi_{461..468} (8 alike) : DataTypeConversion  OutDataTypeStr=double
  emi_855 : Subsystem  TreatAsAtomicUnit=on
  emi_857 : If  IfExpression=Inf <= u1  SampleTime=[1 0]
  emi_858 : DataTypeConversion  OutDataTypeStr=double
  cfblk2 : Outport
  wires:
  cfblk5/1 -> cyemi_465/1, cyemi_467/1
  cfblk3/1 -> cfblk2/1
  cyemi_461/1 -> cfblk3/1
  cfblk1/1 -> cyemi_461/1
  cyemi_462/1 -> cfblk3/2
  cfblk6/1 -> cyemi_462/1
  cyemi_463/1 -> cfblk4/1
  cfblk8/1 -> cyemi_463/1, emi_858/1
  cyemi_464/1 -> cfblk5/1
  cfblk4/1 -> cyemi_464/1
  cyemi_465/1 -> cfblk6/1
  cyemi_466/1 -> cfblk6/2
  cyemi_468/1 -> cfblk8/1
  cyemi_467/1 -> cfblk7/1(emi_853)
  cfblk7/1(emi_854) -> cyemi_468/1, cyemi_466/1
  emi_857/1 -> cfblk7/Action
  emi_857/2 -> emi_855/Action
  emi_858/1 -> emi_857/1

== system sampleModel7126_pp_1_1/cfblk261/cfblk14 ==
  cfblk1 : Inport
  cfblk5 : Inport  Port=2
  Action Port : ActionPort  ActionType=else
  cfblk3 : simulink/Discrete/Difference  ICPrevInput=0.0  OutMin=[]  OutMax=[]  OutDataTypeStr=double  OutputDataTypeScalingMode=double  OutDataType=fixdt(1, 16)  OutScaling=2^-10  DoSatur=off
  cfblk4 : simulink/Discrete/Tapped Delay  vinit=0.0  samptime=-1  NumDelays=1  DelayOrder=Oldest  includeCurrent=off
  cyemi_471 : DataTypeConversion  OutDataTypeStr=double
  cyemi_472 : DataTypeConversion  OutDataTypeStr=double
  cfblk2 : Outport
  cfblk6 : Outport  Port=2
  cfblk7 : Outport  Port=3
  wires:
  cfblk1/1 -> cfblk2/1
  cfblk4/1 -> cfblk7/1
  cfblk5/1 -> cfblk6/1, cyemi_471/1
  cyemi_471/1 -> cfblk3/1
  cyemi_472/1 -> cfblk4/1
  cfblk3/1 -> cyemi_472/1

== system sampleModel7126_pp_1_1/cfblk261/cfblk15 ==
  emi_1964 : Inport
  Action Port : ActionPort  ActionType=then
  cfblk15 : Delay
  emi_1965 : Outport
  wires:
  emi_1964/1 -> cfblk15/1
  cfblk15/1 -> emi_1965/1

== system sampleModel7126_pp_1_1/cfblk261/cfblk8 ==
  emi_1971 : Inport
  Action Port : ActionPort  ActionType=then
  cfblk8 : DiscreteZeroPole  Poles=[0 0.5]  Gain=1  SampleTime=-1
  emi_1972 : Outport
  wires:
  emi_1971/1 -> cfblk8/1
  cfblk8/1 -> emi_1972/1

== system sampleModel7126_pp_1_1/cfblk261/cfblk9 ==
  emi_2194 : Inport
  Action Port : ActionPort  ActionType=then
  cfblk9 : simulink/Continuous/PID Controller  Controller=PID  TimeDomain=Discrete-time  SampleTime=-1  IntegratorMethod=Forward Euler  FilterMethod=Forward Euler  Form=Parallel  UseFilter=on  ControllerParametersSource=internal  P=1  I=1  D=0  N=100  InitialConditionSource=internal  InitialConditionForIntegrator=0  InitialConditionForFilter=0  ExternalReset=none  LimitOutput=off  UpperSaturationLimit=inf  LowerSaturationLimit=-inf  LinearizeAsGain=off  AntiWindupMode=none  Kb=1  TrackingMode=off  Kt=1  PParamMin=[]  PParamMax=[]  IParamMin=[]  IParamMax=[]  DParamMin=[]  DParamMax=[]  NParamMin=[]  NParamMax=[]  KbParamMin=[]  KbParamMax=[]  KtParamMin=[]  KtParamMax=[]  POutMin=[]  POutMax=[]  IOutMin=[]  IOutMax=[]  DOutMin=[]  DOutMax=[]  NOutMin=[]  NOutMax=[]  KbOutMin=[]  KbOutMax=[]  KtOutMin=[]  KtOutMax=[]  IntegratorOutMin=[]  IntegratorOutMax=[]  FilterOutMin=[]  FilterOutMax=[]  SumOutMin=[]  SumOutMax=[]  SumI1OutMin=[]  SumI1OutMax=[]  SumI2OutMin=[]  SumI2OutMax=[]  SumI3OutMin=[]  SumI3OutMax=[]  SumDOutMin=[]  SumDOutMax=[]  SaturationOutMin=[]  SaturationOutMax=[]  IntegratorContinuousStateAttributes=''  IntegratorStateMustResolveToSignalObject=off  IntegratorRTWStateStorageClass=Auto  FilterContinuousStateAttributes=''  FilterStateMustResolveToSignalObject=off  FilterRTWStateStorageClass=Auto  DifferentiatorICPrevScaledInput=0  DifferentiatorOutMin=[]  DifferentiatorOutMax=[]  FilterDiffOutCoefMin=[]  FilterDiffOutCoefMax=[]  SumDenOutMin=[]  SumDenOutMax=[]  SumNumOutMin=[]  SumNumOutMax=[]  ReciprocalOutMin=[]  ReciprocalOutMax=[]  DivideOutMin=[]  DivideOutMax=[]  TunerSelectOption=Transfer Function Based (PID Tuner App)
  emi_2195 : Outport
  wires:
  emi_2194/1 -> cfblk9/1
  cfblk9/1 -> emi_2195/1

== system sampleModel7126_pp_1_1/cfblk261/emi_1966 ==
  Action Port : ActionPort  ActionType=else
  emi_1967 : Assertion

== system sampleModel7126_pp_1_1/cfblk261/emi_1973 ==
  Action Port : ActionPort  ActionType=else
  emi_1974 : Assertion

== system sampleModel7126_pp_1_1/cfblk261/emi_2196 ==
  Action Port : ActionPort  ActionType=else
  emi_2197 : Assertion

== system sampleModel7126_pp_1_1/cfblk262/cfblk4 ==
  emi_474 : Inport
  Action Port : ActionPort  ActionType=then
  cfblk4 : DiscreteIntegrator  SampleTime=-1  OutDataTypeStr=double  ICPrevOutput=DiscIntNeverNeededParam  ICPrevScaledInput=DiscIntNeverNeededParam
  emi_475 : Outport
  wires:
  emi_474/1 -> cfblk4/1
  cfblk4/1 -> emi_475/1

== system sampleModel7126_pp_1_1/cfblk262/cfblk5 ==
  emi_50 : Inport
  emi_51 : Inport  Port=2
  Action Port : ActionPort  ActionType=then
  cfblk5 : Delay  DelayLengthSource=Input port
      settings: InputPortMap=u0,p1
  emi_52 : Outport
  wires:
  emi_50/1 -> cfblk5/1
  emi_51/1 -> cfblk5/2
  cfblk5/1 -> emi_52/1

== system sampleModel7126_pp_1_1/cfblk262/cfblk6 ==
  emi_330 : Inport
  Action Port : ActionPort  ActionType=then
  cfblk6 : simulink/Discrete/Transfer Fcn Real Zero  ZeroZ=0.75  ICPrevInput=0.0  DoSatur=off
      settings: SourceProductName=Simulink  SourceProductBaseCode=SL
  emi_331 : Outport
  wires:
  emi_330/1 -> cfblk6/1
  cfblk6/1 -> emi_331/1

== system sampleModel7126_pp_1_1/cfblk262/emi_332 ==
  Action Port : ActionPort  ActionType=else
  emi_333 : Assertion

== system sampleModel7126_pp_1_1/cfblk262/emi_476 ==
  Action Port : ActionPort  ActionType=else
  emi_477 : Assertion

== system sampleModel7126_pp_1_1/cfblk262/emi_53 ==
  Action Port : ActionPort  ActionType=else
  emi_54 : Assertion

== system sampleModel7126_pp_1_1/cfblk263/cfblk15 ==
  cfblk1 : Inport
  cfblk11 : Inport  Port=2
  Action Port : ActionPort  ActionType=then
  cfblk10 : Subsystem  TreatAsAtomicUnit=on
  cfblk13 : Delay
  cfblk3 : Subsystem  TreatAsAtomicUnit=on
  cfblk4 : UnitDelay  SampleTime=-1
  cfblk5 : simulink/Discrete/Tapped Delay  vinit=0.0  samptime=-1  NumDelays=1  DelayOrder=Oldest  includeCurrent=off
  cfblk6 : DiscreteFir
  cfblk7 : simulink/Discrete/Transfer Fcn Lead or Lag  PoleZ=0.95  ZeroZ=0.75  ICPrevOutput=0.0  ICPrevInput=0.0  DoSatur=off
      settings: SourceProductName=Simulink  SourceProductBaseCode=SL
  cfblk8 : Subsystem  TreatAsAtomicUnit=on
  cfblk9 : DiscreteStateSpace  SampleTime=-1
  cyemi_{502..503,505..508,510..511} (8 alike) : DataTypeConversion  OutDataTypeStr=double
  cyemi_504 : DataTypeConversion  OutDataTypeStr=fixdt('ufix32_En8')
  cyemi_509 : DataTypeConversion  OutDataTypeStr=fixdt('ufix32_En8')
  emi_741 : Subsystem  TreatAsAtomicUnit=on
  emi_743 : If  IfExpression=Inf <= u1
  emi_744 : DataTypeConversion  OutDataTypeStr=double
  emi_784 : Subsystem  TreatAsAtomicUnit=on
  emi_786 : If  IfExpression=Inf <= u1  SampleTime=[1 0]
  emi_787 : DataTypeConversion  OutDataTypeStr=double
  emi_919 : Subsystem  TreatAsAtomicUnit=on
  emi_921 : If  IfExpression=Inf <= u1  SampleTime=[1 0]
  emi_922 : DataTypeConversion  OutDataTypeStr=double
  cfblk2 : Outport
  cfblk12 : Outport  Port=2
  wires:
  cfblk9/1 -> cyemi_502/1, cyemi_507/1
  cfblk4/1 -> cfblk12/1, emi_744/1, emi_787/1, emi_922/1
  cyemi_503/1 -> cfblk13/1
  cfblk7/1 -> cyemi_503/1
  cfblk11/1 -> cyemi_504/1
  cyemi_505/1 -> cfblk4/1
  cyemi_506/1 -> cfblk5/1
  cfblk13/1 -> cyemi_506/1
  cyemi_507/1 -> cfblk6/1
  cyemi_508/1 -> cfblk7/1
  cfblk6/1 -> cyemi_508/1
  cfblk1/1 -> cyemi_510/1
  cyemi_511/1 -> cfblk9/1
  cfblk5/1 -> cyemi_511/1
  cyemi_502/1 -> cfblk10/1(emi_739)
  cfblk10/1(emi_740) -> cfblk2/1
  emi_743/1 -> cfblk10/Action
  emi_743/2 -> emi_741/Action
  emi_744/1 -> emi_743/1
  cyemi_509/1 -> cfblk8/1(emi_781)
  cyemi_510/1 -> cfblk8/2(emi_782)
  cfblk8/1(emi_783) -> cyemi_505/1
  emi_786/1 -> cfblk8/Action
  emi_786/2 -> emi_784/Action
  emi_787/1 -> emi_786/1
  cyemi_504/1 -> cfblk3/1(emi_917)
  cfblk3/1(emi_918) -> cyemi_509/1
  emi_921/1 -> cfblk3/Action
  emi_921/2 -> emi_919/Action
  emi_922/1 -> emi_921/1

== system sampleModel7126_pp_1_1/cfblk263/cfblk16 ==
  cfblk1 : Inport
  cfblk10 : Inport  Port=2
  cfblk11 : Inport  Port=3
  Action Port : ActionPort  ActionType=else
  cfblk3 : Subsystem  TreatAsAtomicUnit=on
  cfblk4 : Subsystem  TreatAsAtomicUnit=on
  cfblk5 : Subsystem  TreatAsAtomicUnit=on
  cfblk6 : Subsystem  TreatAsAtomicUnit=on
  cfblk7 : simulink/Discrete/Difference  ICPrevInput=0.0  OutMin=[]  OutMax=[]  OutDataTypeStr=fixdt('ufix32_En8')  OutputDataTypeScalingMode=Specify via dialog  OutDataType=fixdt('ufix32_En8')  OutScaling=[]  DoSatur=off
  cfblk8 : simulink/Discrete/Difference  ICPrevInput=0.0  OutMin=[]  OutMax=[]  OutDataTypeStr=fixdt('ufix32_En8')  OutputDataTypeScalingMode=Specify via dialog  OutDataType=fixdt('ufix32_En8')  OutScaling=[]  DoSatur=off
  cfblk9 : UnitDelay  SampleTime=-1
  cyemi_515 : DataTypeConversion  OutDataTypeStr=uint8
  cyemi_{516,518..521} (5 alike) : DataTypeConversion  OutDataTypeStr=fixdt('ufix32_En8')
  cyemi_517 : DataTypeConversion  OutDataTypeStr=uint8
  emi_1557 : Subsystem  TreatAsAtomicUnit=on
  emi_1559 : If  IfExpression=0 <= u1
  emi_{681,915,1560,1983} (4 alike) : DataTypeConversion  OutDataTypeStr=fixdt('ufix32_En8')
  emi_1980 : Subsystem  TreatAsAtomicUnit=on
  emi_1982 : If  IfExpression=0 <= u1
  emi_678 : Subsystem  TreatAsAtomicUnit=on
  emi_680 : If  IfExpression=0 <= u1  SampleTime=[1 0]
  emi_912 : Subsystem  TreatAsAtomicUnit=on
  emi_914 : If  IfExpression=0 <= u1  SampleTime=[1 0]
  cfblk2 : Outport
  cfblk12 : Outport  Port=2
  cfblk13 : Outport  Port=3
  wires:
  cfblk11/1 -> cfblk2/1
  cfblk7/1 -> cfblk13/1
  cfblk8/1 -> cyemi_516/1
  cfblk1/1 -> cyemi_517/1
  cyemi_519/1 -> cfblk7/1
  cyemi_520/1 -> cfblk8/1
  cfblk9/1 -> cyemi_520/1, emi_1983/1
  cyemi_521/1 -> cfblk9/1
  cfblk10/1 -> cyemi_521/1
  cyemi_517/1 -> cfblk5/1(emi_676)
  cfblk5/1(emi_677) -> cyemi_515/1
  emi_680/1 -> cfblk5/Action
  emi_680/2 -> emi_678/Action
  emi_681/1 -> emi_680/1
  cyemi_518/1 -> cfblk6/1(emi_910)
  cfblk6/1(emi_911) -> emi_681/1, cfblk12/1
  emi_914/1 -> cfblk6/Action
  emi_914/2 -> emi_912/Action
  emi_915/1 -> emi_914/1
  cyemi_516/1 -> cfblk4/1(emi_1555)
  cfblk4/1(emi_1556) -> cyemi_519/1
  emi_1559/1 -> cfblk4/Action
  emi_1559/2 -> emi_1557/Action
  emi_1560/1 -> emi_1559/1
  cyemi_515/1 -> cfblk3/1(emi_1978)
  cfblk3/1(emi_1979) -> emi_1560/1, emi_915/1, cyemi_518/1
  emi_1982/1 -> cfblk3/Action
  emi_1982/2 -> emi_1980/Action
  emi_1983/1 -> emi_1982/1
